simulink model "BallAndBeam_Workspace"  (R2022b)
settings: Solver=ode4  StartTime=0.0  StopTime=inf  FixedStep=0.001  RelTol=1e-3  EnableMultiTasking=on
model workspace (MAT data in the model file):
  GR = 70
  J_s = 0.00177142857143
  L_b = 0.4255
  R_m = 2.6
  g = 9.81
  k_t = 0.007683
  k_v = 0.006983
  m_b = 0.064
  m_r = 0.1
  mu_v = 0.0001
  r_arm = 0.0254
  r_rod = 0.00158369
  tau_k = 0.03
  tau_s = 0.04
undefined symbols (not defined in the file or in its folder): qc_get_step_size
libraries: quarc_library x4, simulink x1
settings Model: SimulationMode=external  ExtModeTrigDuration=10000  Creator=MLevis  LastModifiedBy=Derek
settings SolverCC: AlgebraicLoopSolver=TrustRegion  PositivePriorityOrder=on
settings DataIOCC: ReturnWorkspaceOutputs=off
settings DebuggingCC: UnconnectedInputMsg=warning  UnconnectedOutputMsg=warning  UnconnectedLineMsg=warning  SFMachineParentedDataDiag=warning  ArithmeticOperatorsInVariantConditions=warning
settings HardwareCC: ProdBitPerLong=64  ProdHWDeviceType=Intel->x86-64 (Mac OS X)
settings ModelReferenceCC: EnableRefExpFcnMdlSchedulingChecks=on
settings SFSimCC: SimUseLocalCustomCode=off  CustomCodeUndefinedFunction=UseInterfaceOnly
settings RTWCC: Description=QUARC Mac x86_64 Target Using Toolchain  SystemTargetFile=quarc_mac_x86_64.tlc  TemplateMakefile=quarc_default_tmf  PostCodeGenCommand=packNGo(buildInfo, 'packType', 'hierarchical')  RTWUseLocalCustomCode=off  Toolchain=QUARC mac_x86_64 | gmake (64-bit Windows)  BuildConfiguration=Faster Runs  DLArmComputeVersion=19.05
settings CodeAppCC: StateflowObjectComments=on
settings STFCustomTargetCC: TargetLangStandard=C99 (ISO)  ConcurrentExecutionCompliant=on  GRTInterface=on  UseToolchainInfoCompliant=on  SystemTargetFile=quarc_mac_x86_64.tlc
settings GRTTargetCC: ParMdlRefBuildCompliant=off  CompOptLevelCompliant=off  CombineOutputUpdateFcns=off  MatFileLogging=off  CPPClassGenCompliant=off  GRTInterface=on  ExtMode=on  ExtModeMexFile=quarc_comm  ExtModeMexArgs='-w -d /tmp -uri %u'
settings ConfigComp: CovMetricSettings=dswe

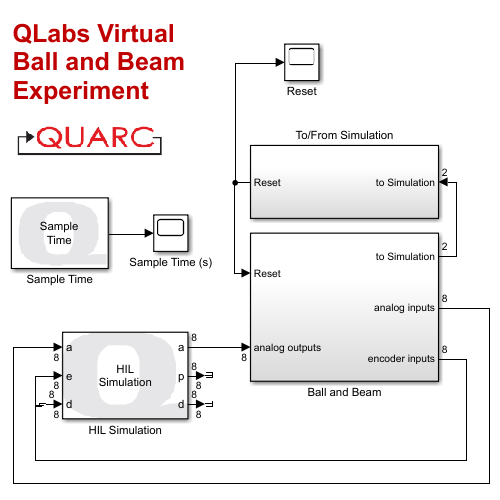
[thumbnail: Simulink's stored preview of the top-level diagram]
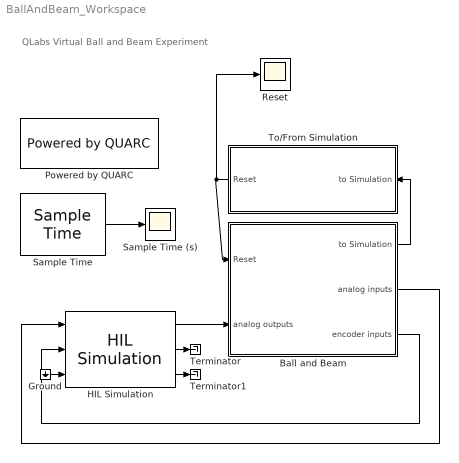
== system BallAndBeam_Workspace ==
  note: QLabs Virtual
      | Ball and Beam
      | Experiment
  Ball and Beam : Subsystem
  Ground : Ground
  HIL Simulation : quarc_library/Data Acquisition/Generic/Configuration/HIL Simulation  uri=tcpip://localhost:18942  board_type=q8_usb  board_id=0  sample_time=qc_get_step_size  active=on  num_clocks=1  num_interrupts=0  num_analog_inputs=8  num_analog_outputs=8  initial_analog=[]  num_digital_io=0  num_digital_inputs=8  num_digital_outputs=8  initial_digital=[]  num_encoder_inputs=8  num_pwm_outputs=8  initial_pwm=[]  other_inputs=[]  other_outputs=[]  initial_other=[]  integer_get_property_codes=[]  double_get_property_codes=[]  string_get_property_codes=[]  integer_set_property_codes=[]  double_set_property_codes=[]  string_set_property_codes=[]  initial_integer_properties=0  initial_double_properties=0  initial_string_properties=[]  max_string_property=80  use_variable_size_strings=off
      settings: SourceProductName=QUARC Targets
  Powered by QUARC : quarc_library/Logos/Powered by QUARC
  Reset : Scope
  Sample Time : quarc_library/Sources/Time/Sample Time  Priority=-99  sample_time=qc_get_step_size
  Sample Time (s) : Scope
  Terminator : Terminator
  Terminator1 : Terminator
  To/From Simulation : Subsystem
  wires:
  Sample Time/1 -> Sample Time (s)/1
  To/From Simulation/1(Reset) -> Reset/1, Ball and Beam/1(Reset)
  Ball and Beam/2(analog inputs) -> HIL Simulation/1
  Ball and Beam/3(encoder inputs) -> HIL Simulation/2
  HIL Simulation/1 -> Ball and Beam/2(analog outputs)
  Ball and Beam/1(to Simulation) -> To/From Simulation/1(to Simulation)
  Ground/1 -> HIL Simulation/3
  HIL Simulation/2 -> Terminator/1
  HIL Simulation/3 -> Terminator1/1

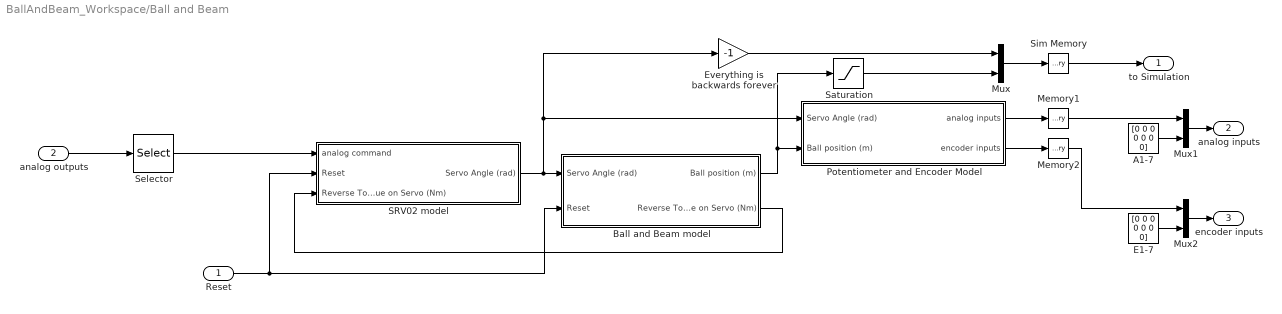
== system BallAndBeam_Workspace/Ball and Beam ==
  Reset : Inport
  analog outputs : Inport  Port=2
  A1-7 : Constant  Value=[0 0 0 0 0 0 0]
  Ball and Beam model : Subsystem
  E1-7 : Constant  Value=[0 0 0 0 0 0 0]  OutDataTypeStr=int32
  Everything is backwards forever : Gain  Gain=-1
  Memory1 : Memory
  Memory2 : Memory
  Mux : Mux  Inputs=2
  Mux1 : Mux  Inputs=2
  Mux2 : Mux  Inputs=2
  Potentiometer and Encoder Model : Subsystem
  SRV02 model : Subsystem
  Saturation : Saturate  UpperLimit=L_b/2-0.015  LowerLimit=-L_b/2+0.015
  Selector : Selector  InputPortWidth=8  IndexOptions=Index vector (dialog)  Indices=[1]  OutputSizes=1
  Sim Memory : Memory  InitialCondition=[0 0]
  to Simulation : Outport  VectorParamsAs1DForOutWhenUnconnected=off
  analog inputs : Outport  Port=2  VectorParamsAs1DForOutWhenUnconnected=off
  encoder inputs : Outport  Port=3  VectorParamsAs1DForOutWhenUnconnected=off
  wires:
  Ball and Beam model/2(Reverse Torque on Servo (Nm)) -> SRV02 model/3(Reverse Torque on Servo (Nm))
  SRV02 model/1(Servo Angle (rad)) -> Everything is backwards forever/1, Potentiometer and Encoder Model/1(Servo Angle (rad)), Ball and Beam model/1(Servo Angle (rad))
  Potentiometer and Encoder Model/2(encoder inputs) -> Memory2/1
  Potentiometer and Encoder Model/1(analog inputs) -> Memory1/1
  analog outputs/1 -> Selector/1
  Ball and Beam model/1(Ball position (m)) -> Saturation/1, Potentiometer and Encoder Model/2(Ball position (m))
  Mux/1 -> Sim Memory/1
  Reset/1 -> Ball and Beam model/2(Reset), SRV02 model/2(Reset)
  Sim Memory/1 -> to Simulation/1
  Memory1/1 -> Mux1/1
  Memory2/1 -> Mux2/1
  Mux1/1 -> analog inputs/1
  Mux2/1 -> encoder inputs/1
  E1-7/1 -> Mux2/2
  Selector/1 -> SRV02 model/1(analog command)
  A1-7/1 -> Mux1/2
  Everything is backwards forever/1 -> Mux/1
  Saturation/1 -> Mux/2

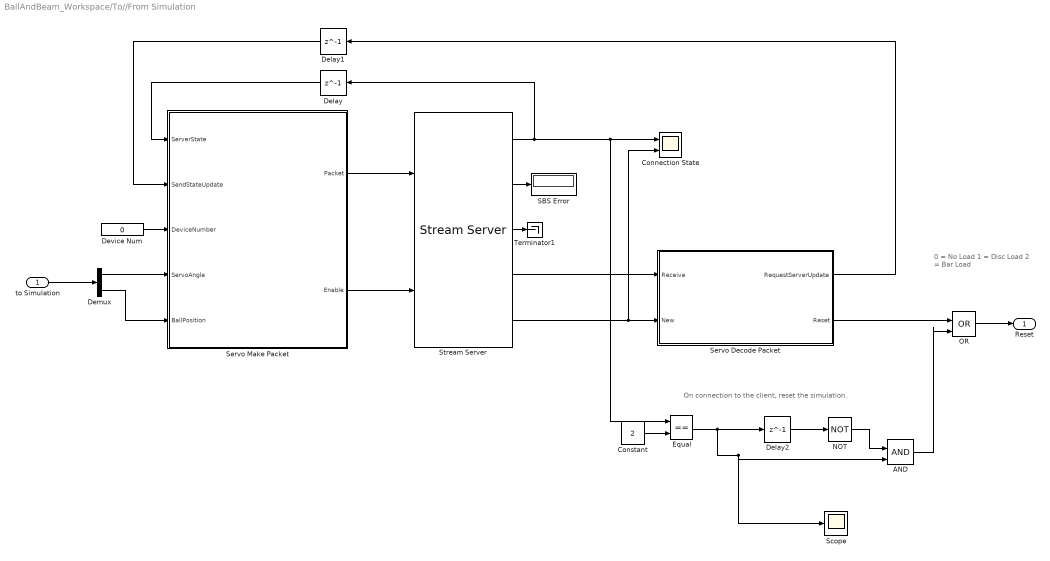
== system BallAndBeam_Workspace/To//From Simulation ==
  note: On connection to the client, reset the simulation.
  note: 0 = No Load
      | 1 = Disc Load
      | 2 = Bar Load
  to Simulation : Inport
  AND : Logic  IconShape=distinctive  AllPortsSameDT=off  OutDataTypeStr=boolean
  "Connection State " : Scope  NumInputPorts=2
  Constant : Constant  Value=2
  Delay : Delay  DelayLength=1
  Delay1 : Delay  DelayLength=1
  Delay2 : Delay  DelayLength=1
  Demux : Demux  Outputs=2
  Device Num : Constant  Value=0
  Equal : RelationalOperator  Operator===  OutDataTypeStr=boolean  RndMeth=Simplest  InputSameDT=off
  NOT : Logic  Operator=NOT  IconShape=distinctive  AllPortsSameDT=off  OutDataTypeStr=boolean
  OR : Logic  Operator=OR  IconShape=distinctive  AllPortsSameDT=off  OutDataTypeStr=boolean
  SBS Error : Display
  Scope : Scope
  Servo Decode Packet : MATLAB Function  TreatAsAtomicUnit=on
  Servo Make Packet : MATLAB Function  TreatAsAtomicUnit=on
  Stream Server : quarc_library/Communications/Basic/Stream Server  uri_source=Specify via dialog (do not evaluate)  uri=tcpip://remotehost:18001?nagle='off'  send_buffer_size=65537  receive_buffer_size=65537  byte_order=little endian (Intel - LSB first)  optimization=Minimum latency  send_options=Send all data  receive_options=Receive all data  default_value=[0]  sample_time=qc_get_step_size  active=on  implementation=Use blocking I/O in a separate thread  send_fifo_size=3  receive_fifo_size=3  send_priority=0  receive_priority=0  send_dimensions=on  receive_dimensions=on  max_dimensions=65537  data_type=uint8  type_expr=BusObject
      settings: AttributesFormatString="\"tcpip://remotehost:18001?nagle='off'\""
  Terminator1 : Terminator
  Reset : Outport  VectorParamsAs1DForOutWhenUnconnected=off
  wires:
  Stream Server/2 -> SBS Error/1
  Servo Decode Packet/2(Reset) -> OR/1
  Delay1/1 -> Servo Make Packet/2(SendStateUpdate)
  Delay/1 -> Servo Make Packet/1(ServerState)
  Device Num/1 -> Servo Make Packet/3(DeviceNumber)
  Stream Server/3 -> Terminator1/1
  Stream Server/1 -> Delay/1, Equal/1, "Connection State "/1
  Servo Make Packet/2(Enable) -> Stream Server/2
  Servo Decode Packet/1(RequestServerUpdate) -> Delay1/1
  Stream Server/5 -> "Connection State "/2, Servo Decode Packet/2(New)
  Servo Make Packet/1(Packet) -> Stream Server/1
  Stream Server/4 -> Servo Decode Packet/1(Receive)
  to Simulation/1 -> Demux/1
  Demux/1 -> Servo Make Packet/4(ServoAngle)
  Demux/2 -> Servo Make Packet/5(BallPosition)
  Constant/1 -> Equal/2
  Delay2/1 -> NOT/1
  Equal/1 -> Scope/1, AND/2, Delay2/1
  NOT/1 -> AND/1
  OR/1 -> Reset/1
  AND/1 -> OR/2

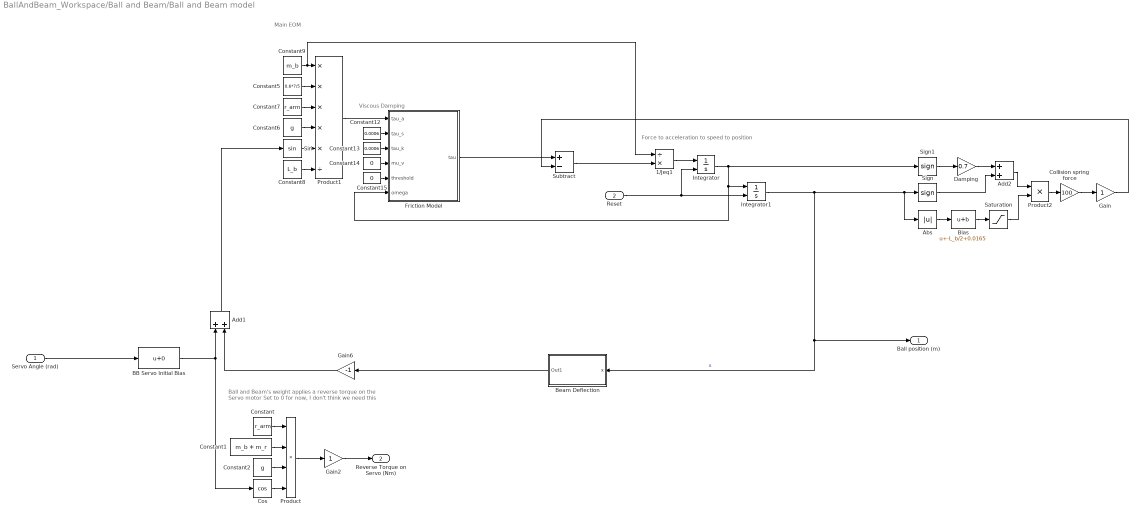
== system BallAndBeam_Workspace/Ball and Beam/Ball and Beam model ==
  note: Ball and Beam's weight applies a
      | reverse torque on the Servo motor
      | Set to 0 for now, I don't think we need this
  note: Force to acceleration to speed to position
  note: Viscous Damping
  note: Main EOM
  Servo Angle (rad) : Inport
  Reset : Inport  Port=2
  1/Jeq1 : Product  Inputs=/*
  Abs : Abs  SaturateOnIntegerOverflow=off
  Add1 : Sum
  Add2 : Sum
  BB Servo Initial Bias : Bias  SaturateOnIntegerOverflow=off
  Beam Deflection : Subsystem
  Bias : Bias  Bias=-L_b/2+0.0165  SaturateOnIntegerOverflow=off
  Collision spring force : Gain  Gain=100
  Constant : Constant  Value=r_arm
  Constant1 : Constant  Value=m_b + m_r  VectorParams1D=off
  Constant12 : Constant  Value=0.0006
  Constant13 : Constant  Value=0.0006
  Constant14 : Constant  Value=0
  Constant15 : Constant  Value=0
  Constant2 : Constant  Value=g
  Constant5 : Constant  Value=0.6*7/5
  Constant6 : Constant  Value=g
  Constant7 : Constant  Value=r_arm
  Constant8 : Constant  Value=L_b
  Constant9 : Constant  Value=m_b
  Cos : Trigonometry  Operator=cos
  Damping : Gain  Gain=0.7
  "Friction Model " : MATLAB Function  TreatAsAtomicUnit=on
  Gain : Gain
  Gain2 : Gain
  Gain6 : Gain  Gain=-1
  Integrator : Integrator  ExternalReset=rising
  Integrator1 : Integrator  ExternalReset=rising  UpperSaturationLimit=L_b/2-0.05  LowerSaturationLimit=-L_b/2+0.05
  Product : Product  Inputs=4
  Product1 : Product  Inputs=*****/
  Product2 : Product
  Saturation : Saturate  UpperLimit=1  LowerLimit=0
  Sign : Signum
  Sign1 : Signum
  Sin : Trigonometry
  Subtract : Sum  Inputs=+-
  Ball position (m) : Outport  VectorParamsAs1DForOutWhenUnconnected=off
  Reverse Torque on Servo (Nm) : Outport  Port=2  VectorParamsAs1DForOutWhenUnconnected=off
  wires:
  Product1/1 -> "Friction Model "/1(tau_a)
  Constant7/1 -> Product1/3
  Constant12/1 -> "Friction Model "/2(tau_s)
  "Friction Model "/1(tau) -> Subtract/1
  Abs/1 -> Bias/1
  Constant9/1 -> 1/Jeq1/1, Product1/1
  Constant6/1 -> Product1/4
  Constant14/1 -> "Friction Model "/4(mu_v)
  1/Jeq1/1 -> Integrator/1
  Constant13/1 -> "Friction Model "/3(tau_k)
  Subtract/1 -> 1/Jeq1/2
  Integrator/1 -> "Friction Model "/6(omega), Integrator1/1, Sign1/1
  Integrator1/1 -> Sign/1, Abs/1, Beam Deflection/1(x), Ball position (m)/1  "x"
  Constant15/1 -> "Friction Model "/5(threshold)
  Sin/1 -> Product1/5
  Constant8/1 -> Product1/6
  Constant5/1 -> Product1/2
  BB Servo Initial Bias/1 -> Cos/1, Add1/1
  Gain2/1 -> Reverse Torque on Servo (Nm)/1
  Constant2/1 -> Product/3
  Cos/1 -> Product/4
  Constant/1 -> Product/1
  Constant1/1 -> Product/2
  Product/1 -> Gain2/1
  Servo Angle (rad)/1 -> BB Servo Initial Bias/1
  Reset/1 -> Integrator1/2, Integrator/2
  Add1/1 -> Sin/1
  Beam Deflection/1(Out1) -> Gain6/1
  Gain6/1 -> Add1/2
  Bias/1 -> Saturation/1
  Gain/1 -> Subtract/2
  Sign/1 -> Add2/2
  Product2/1 -> Collision spring force/1
  Collision spring force/1 -> Gain/1
  Sign1/1 -> Damping/1
  Damping/1 -> Add2/1
  Add2/1 -> Product2/1
  Saturation/1 -> Product2/2

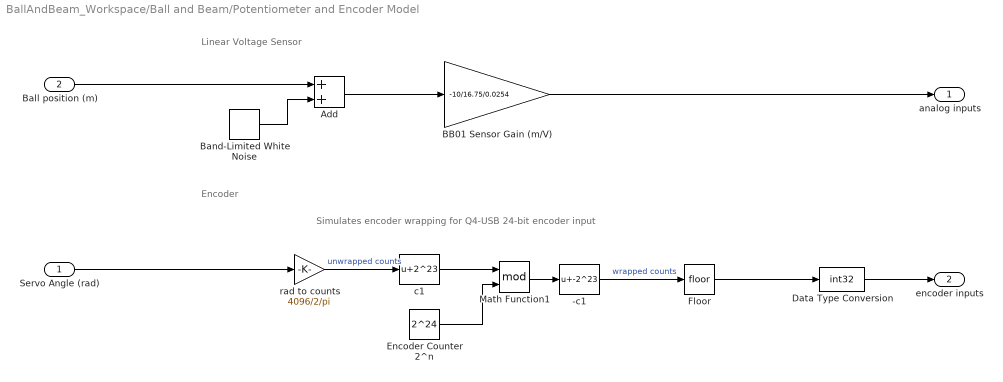
== system BallAndBeam_Workspace/Ball and Beam/Potentiometer and Encoder Model ==
  note: Linear Voltage Sensor
  note: Encoder
  note: Simulates encoder wrapping for Q4-USB 24-bit encoder input
  Servo Angle (rad) : Inport
  Ball position (m) : Inport  Port=2
  -c1 : Bias  Bias=-2^23  SaturateOnIntegerOverflow=off
  Add : Sum
  BB01 Sensor Gain (m/V) : Gain  Gain=-10/16.75/0.0254
  Band-Limited White Noise : simulink/Sources/Band-Limited White Noise  Cov=0.00000000001  Ts=qc_get_step_size  seed=randi(10000,1)
  Data Type Conversion : DataTypeConversion  OutDataTypeStr=int32  SaturateOnIntegerOverflow=off  RndMeth=Floor
  Encoder Counter 2^n : Constant  Value=2^24
  Floor : Rounding
  Math Function1 : Math  Operator=mod  SignedPower=on
  c1 : Bias  Bias=2^23  SaturateOnIntegerOverflow=off
  rad to counts : Gain  Gain=4096/2/pi
  analog inputs : Outport  VectorParamsAs1DForOutWhenUnconnected=off
  encoder inputs : Outport  Port=2  VectorParamsAs1DForOutWhenUnconnected=off
  wires:
  Floor/1 -> Data Type Conversion/1
  Data Type Conversion/1 -> encoder inputs/1
  Servo Angle (rad)/1 -> rad to counts/1
  -c1/1 -> Floor/1  "wrapped counts"
  rad to counts/1 -> c1/1  "unwrapped counts"
  Encoder Counter 2^n/1 -> Math Function1/2
  c1/1 -> Math Function1/1
  Math Function1/1 -> -c1/1
  Add/1 -> BB01 Sensor Gain (m/V)/1
  BB01 Sensor Gain (m/V)/1 -> analog inputs/1
  Band-Limited White Noise/1 -> Add/2
  Ball position (m)/1 -> Add/1

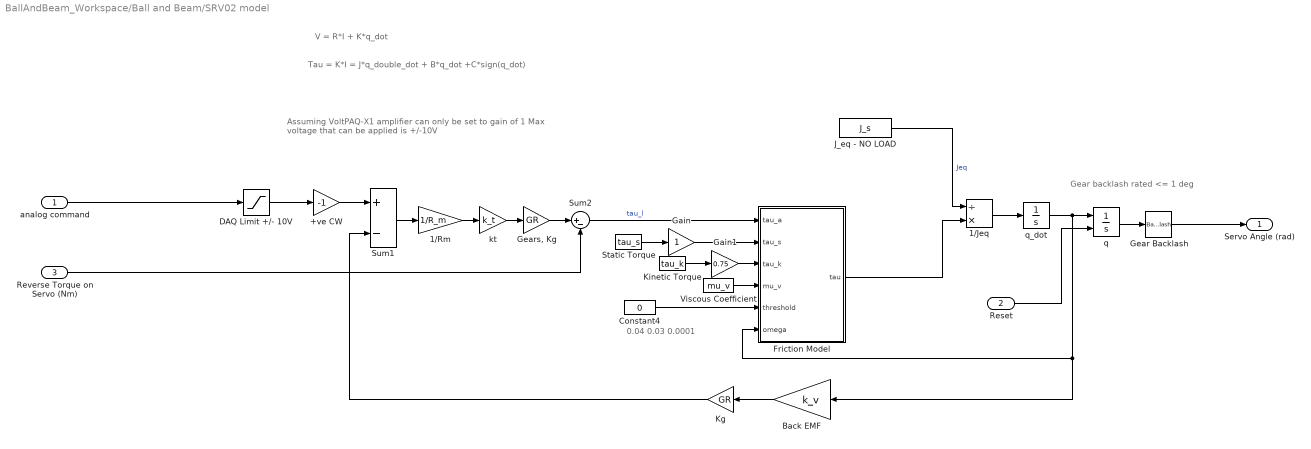
== system BallAndBeam_Workspace/Ball and Beam/SRV02 model ==
  note: Tau = K*I = J*q_double_dot + B*q_dot +C*sign(q_dot)
  note: 0.04
      | 0.03
      | 0.0001
  note: Assuming VoltPAQ-X1 amplifier can only be set to gain of 1
      | Max voltage that can be applied is +/-10V
  note: Gear backlash rated <= 1 deg
  note: V = R*I + K*q_dot
  analog command : Inport
  Reset : Inport  Port=2
  Reverse Torque on Servo (Nm) : Inport  Port=3
  +ve CW : Gain  Gain=-1
  1/Jeq : Product  Inputs=/*
  1/Rm : Gain  Gain=1/R_m
  Back EMF : Gain  Gain=k_v
  Constant4 : Constant  Value=0
  DAQ Limit +/- 10V : Saturate  UpperLimit=10  LowerLimit=-10
  Friction Model : MATLAB Function  TreatAsAtomicUnit=on
  Gain : Gain
  Gain1 : Gain  Gain=0.75
  Gear Backlash : Backlash  BacklashWidth=1/180*pi
  "Gears, Kg" : Gain  Gain=GR
  J_eq - NO LOAD : Constant  Value=J_s
  Kg : Gain  Gain=GR
  Kinetic Torque : Constant  Value=tau_k
  Static Torque : Constant  Value=tau_s
  Sum1 : Sum  Inputs=+-
  Sum2 : Sum  Inputs=|+-
  Viscous Coefficient : Constant  Value=mu_v
  kt : Gain  Gain=k_t
  q : Integrator  ExternalReset=either  LimitOutput=on  UpperSaturationLimit=56*pi/180  LowerSaturationLimit=-56*pi/180
  q_dot : Integrator
  Servo Angle (rad) : Outport  VectorParamsAs1DForOutWhenUnconnected=off
  wires:
  q_dot/1 -> Back EMF/1, Friction Model/6(omega), q/1
  Kinetic Torque/1 -> Gain1/1
  Sum2/1 -> Friction Model/1(tau_a)  "tau_l"
  J_eq - NO LOAD/1 -> 1/Jeq/1  "Jeq"
  q/1 -> Gear Backlash/1
  "Gears, Kg"/1 -> Sum2/1
  Constant4/1 -> Friction Model/5(threshold)
  1/Jeq/1 -> q_dot/1
  Static Torque/1 -> Gain/1
  Kg/1 -> Sum1/2
  Friction Model/1(tau) -> 1/Jeq/2
  Gear Backlash/1 -> Servo Angle (rad)/1
  Viscous Coefficient/1 -> Friction Model/4(mu_v)
  Back EMF/1 -> Kg/1
  Sum1/1 -> 1/Rm/1
  DAQ Limit +/- 10V/1 -> +ve CW/1
  kt/1 -> "Gears, Kg"/1
  +ve CW/1 -> Sum1/1
  1/Rm/1 -> kt/1
  Reverse Torque on Servo (Nm)/1 -> Sum2/2
  Reset/1 -> q/2
  analog command/1 -> DAQ Limit +/- 10V/1
  Gain/1 -> Friction Model/2(tau_s)
  Gain1/1 -> Friction Model/3(tau_k)

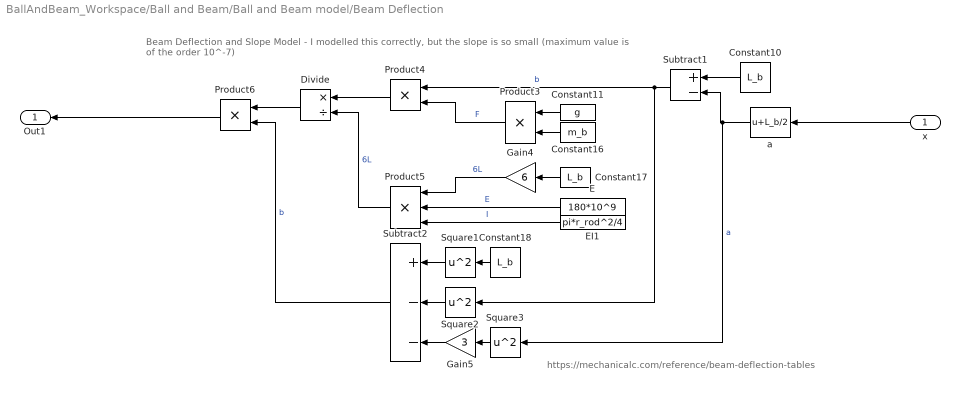
== system BallAndBeam_Workspace/Ball and Beam/Ball and Beam model/Beam Deflection ==
  note: Beam Deflection and Slope Model - I modelled this correctly, but the slope is so small (maximum value is of the order 10^-7)
  note: https://mechanicalc.com/reference/beam-deflection-tables
  x : Inport
  Constant10 : Constant  Value=L_b
  Constant11 : Constant  Value=g
  Constant16 : Constant  Value=m_b
  Constant17 : Constant  Value=L_b
  Constant18 : Constant  Value=L_b
  Divide : Product  Inputs=*/
  E : Constant  Value=180*10^9
  EI1 : Constant  Value=pi*r_rod^2/4
  Gain4 : Gain  Gain=6
  Gain5 : Gain  Gain=3
  Product3 : Product
  Product4 : Product
  Product5 : Product  Inputs=3
  Product6 : Product
  Square1 : Math  Operator=square  SignedPower=on
  Square2 : Math  Operator=square  SignedPower=on
  Square3 : Math  Operator=square  SignedPower=on
  Subtract1 : Sum  Inputs=+-
  Subtract2 : Sum  Inputs=+--
  a : Bias  Bias=L_b/2  SaturateOnIntegerOverflow=off
  Out1 : Outport  VectorParamsAs1DForOutWhenUnconnected=off
  wires:
  Subtract1/1 -> Square2/1, Product4/1  "b"
  Constant18/1 -> Square1/1
  Square3/1 -> Gain5/1
  EI1/1 -> Product5/3  "I"
  Constant10/1 -> Subtract1/1
  Square2/1 -> Subtract2/2
  Subtract2/1 -> Product6/2  "b"
  Divide/1 -> Product6/1
  Product4/1 -> Divide/1
  Constant17/1 -> Gain4/1
  Square1/1 -> Subtract2/1
  Product5/1 -> Divide/2  "6L"
  E/1 -> Product5/2  "E"
  Product6/1 -> Out1/1
  Product3/1 -> Product4/2  "F"
  a/1 -> Square3/1, Subtract1/2  "a"
  Gain4/1 -> Product5/1  "6L"
  Gain5/1 -> Subtract2/3
  Constant16/1 -> Product3/2
  Constant11/1 -> Product3/1
  x/1 -> a/1

== matlab function BallAndBeam_Workspace/To//From Simulation/Servo Make Packet ==
  settings: updateMethod=DISCRETE  sampleTime=qc_get_step_size
  data: Packet output size=65537; ServerState input; SendStateUpdate input; Enable output; DeviceNumber input; ServoAngle input; BallPosition input
function [Packet,Enable] = BB01MakePacket(ServerState, SendStateUpdate, DeviceNumber, ServoAngle, BallPosition) 

% Be sure to set the maximum signal size of the variable size Packet port 
% in Simulink->Edit Data of the editor window.  Size should be 65537 or
% larger to ensure that the stream server generates a 4 byte packet size.

%% Setup
persistent LastServerState;

if isempty(LastServerState)
    LastServerState = uint8(0);
end

Enable = 0;
Packet = uint8([]);

%% On connection
if ((ServerState == 2) && (LastServerState ~= 2))
    Packet = BBeamMakeCommandStateContainer(DeviceNumber, ServoAngle, BallPosition); 
    %%Packet = [Packet; MakeModeRequestContainer(42, DeviceNumber)];
end

%% Send new State Container
% Previous state processed, send a new one
if (SendStateUpdate)
    Packet = BBeamMakeCommandStateContainer(DeviceNumber, ServoAngle, BallPosition); 
end

%% Transmit
% If we have data to send, enable the transmit
PacketLength = length(Packet);

if (PacketLength > 0)
    % Add magic byte.  This is just for error handling and isn't typically
    % required in simulink, but useful in lower-level languages like Python
    Packet = [uint8(123); Packet];
    
    Enable = 1; 
end


LastServerState = ServerState;

== matlab function BallAndBeam_Workspace/Ball and Beam/Ball and Beam model/Friction Model  ==
  data: tau_a input; tau output; tau_s input; tau_k input; mu_v input; threshold input; omega input
function tau = fcn(tau_a, tau_s, tau_k, mu_v, threshold, omega)

% Friction Model:
% tau           - output torque
% tau_a         - applied torque
% tau_s         - static friction torque
% tau_k         - kinetic friction torque
% tau_v         - viscous friction torque
% threshold     - threshold under which you want omega to be considered 0
% omega         - angular speed

% v1.0 Murtaza Bohra
not_moving = 0;
if abs(omega) <= threshold
    not_moving = 1;
end

if (abs(tau_a) < tau_s)&&(not_moving)
    tau = 0;
else
    tau = tau_a - tau_k*sign(omega) - mu_v*omega;
end

== matlab function BallAndBeam_Workspace/To//From Simulation/Servo Decode Packet ==
  data: Receive input size=65537; RequestServerUpdate output; New input; Reset output
function [RequestServerUpdate, Reset] = BB01DecodePacket(Receive, New)

%% Setup

% Need to assign outputs here even though they are reassigned at the end
% since matlab can't determine the signal widths
Reset = 0;
RequestServerUpdate = 0;

PacketSize = length(Receive);

% Packet > 0, new data, and magic number in first index
if ((PacketSize > 0) && (New == 1) && (Receive(1) == uint8(123)))
    
    %skip magic number
    Index = int32(2);
    
    while(Index <= PacketSize)
       
        %% Get container details
        ContainerSize = typecast(uint8(flip(Receive(Index:Index+3))), 'int32');
        DeviceID = typecast(uint8(flip(Receive(Index+4:Index+7))), 'int32');
        DeviceNum = typecast(uint8(flip(Receive(Index+8:Index+11))), 'int32');
        DeviceFunction = uint8(Receive(Index+12));
        PayloadStart = Index+13;
        PayloadEnd = Index+ContainerSize-1;
        
        %% Pass container to appropriate decoding function
        if (DeviceID == 42) %is this a BB01 container?
            
            if (DeviceFunction == 11) %UE4 State Response
                RequestServerUpdate = 1;
            end
        
        elseif (DeviceID == 1001) %Simulink notification
            if (DeviceFunction == 200) %Reset button
                Reset = 1;
            end
        end
        
        
        
        %% Process next container if any data is left.
        Index = Index+ContainerSize;
    end


end

== matlab function BallAndBeam_Workspace/Ball and Beam/SRV02 model/Friction Model ==
  data: tau_a input; tau output; tau_s input; tau_k input; mu_v input; threshold input; omega input
function tau = fcn(tau_a, tau_s, tau_k, mu_v, threshold, omega)

% Friction Model:
% tau           - output torque
% tau_a         - applied torque
% tau_s         - static friction torque
% tau_k         - kinetic friction torque
% tau_v         - viscous friction torque
% threshold     - threshold under which you want omega to be considered 0
% omega         - angular speed

% v1.0 Murtaza Bohra
not_moving = 0;
if abs(omega) <= threshold
    not_moving = 1;
end

if (abs(tau_a) < tau_s)&&(not_moving)
    tau = 0;
else
    tau = tau_a - tau_k*sign(omega) - mu_v*omega;
end
